simulink model "operation_ex"  (R2014a)
settings: Solver=ode45  SolverMode=SingleTasking  StartTime=0.0  StopTime=10.0  RelTol=1e-3
settings Model: CovMetricSettings=dwe  CovHtmlReporting=off  covSaveCumulativeToWorkspaceVar=off  CovSaveSingleToWorkspaceVar=off  CovExternalEMLEnable=on  CovSFcnEnable=on  Creator=lenovo  LastModifiedBy=DELL
settings DataIOCC: LimitDataPoints=off  SaveFormat=StructureWithTime
settings DebuggingCC: MergeDetectMultiDrivingBlocksExec=error  SolverPrmCheckMsg=none  FrameProcessingCompatibilityMsg=error  SFUnexpectedBacktrackingDiag=error  SFNoUnconditionalDefaultTransitionDiag=error
settings HardwareCC: ProdBitPerPointer=64  ProdLargestAtomicFloat=Float  ProdIntDivRoundTo=Zero  ProdEndianess=LittleEndian  ProdHWDeviceType=Specified
settings ModelReferenceCC: PropagateSignalLabelsOutOfModel=on
settings GRTTargetCC: TargetLangStandard=C99 (ISO)

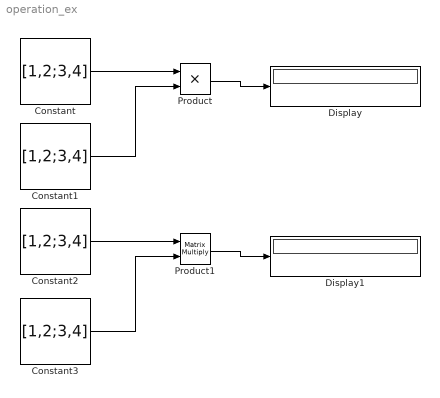
== system operation_ex ==
  Constant{,1..3} (4 alike) : Constant  Value=[1,2;3,4]
  Display : Display
  Display1 : Display
  Product : Product
  Product1 : Product  Multiplication=Matrix(*)
  wires:
  Constant/1 -> Product/1
  Constant2/1 -> Product1/1
  Constant3/1 -> Product1/2
  Constant1/1 -> Product/2
  Product/1 -> Display/1
  Product1/1 -> Display1/1
